simulink model "untitled5"  (Simulink 7.7)
settings: Solver=ode45  StartTime=0.0  StopTime=10.0  RelTol=1e-3
settings Model: Creator=güler  LastModifiedBy=güler

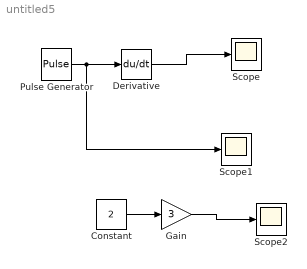
== system untitled5 ==
  Constant : Constant  Value=2
  Derivative : Derivative
  Gain : Gain  Gain=3
  Pulse Generator : DiscretePulseGenerator  PulseType=Time based  Period=1  PulseWidth=50
  Scope : Scope
  Scope1 : Scope
  Scope2 : Scope
      settings: SaveName=ScopeData2
  wires:
  Pulse Generator/1 -> Derivative/1, Scope1/1
  Derivative/1 -> Scope/1
  Gain/1 -> Scope2/1
  Constant/1 -> Gain/1
